simulink model "PubIfDecisionLSM_MDL"  (R2020b)
settings: configuration reference "DspaceConfig" (kept outside this file)
PostLoadFcn:
  | if any(exist('dsrtsu_mdlpostloadfcn', 'file') ~= 0), dsrtsu_mdlpostloadfcn('Execute', bdroot); end
InitFcn:
  | , if any(exist('rtifpga_mdlclblib', 'file') ~= 0), rtifpga_mdlclblib('Init', bdroot); end,
  | , if any(exist('dsmpb_private', 'file') ~= 0), dsmpb_private('dsmpb_mdlclblib', 'Init', bdroot); end,
values from neighbouring files (symbols this model uses):
  P_LSM_ALC_Enable = 0.0    [LSM_Parameter.sldd]
  P_LSM_AwayEdge_offset = 0.1    [LSM_Parameter.sldd]
  P_LSM_CentValidErr = 1.0    [LSM_Parameter.sldd]
  P_LSM_DOP_C0_EN_Limit = 0.8    [LSM_Parameter.sldd]
  P_LSM_DOP_C0_out_Limit = 2.0    [LSM_Parameter.sldd]
  P_LSM_DOP_C1_EN_Limit : value not decoded    [LSM_Parameter.sldd]
  P_LSM_DOP_C1_out_Limit : value not decoded    [LSM_Parameter.sldd]
  P_LSM_DOP_C1AndC2_Lim_X : value not decoded    [LSM_Parameter.sldd]
  P_LSM_DOP_C2_EN_Limit : value not decoded    [LSM_Parameter.sldd]
  P_LSM_DOP_C2_out_Limit : value not decoded    [LSM_Parameter.sldd]
  P_LSM_DOP_In_Pre2Dop_Dis = 1.0    [LSM_Parameter.sldd]
  P_LSM_DOP_Out_Pre2Dop_Dis = 2.0    [LSM_Parameter.sldd]
  P_LSM_DOP_PreDis_X : value not decoded    [LSM_Parameter.sldd]
  P_LSM_DOP_PreDis_Y : value not decoded    [LSM_Parameter.sldd]
  P_LSM_DOPEnableSW = 1.0    [LSM_Parameter.sldd]
  P_LSM_DOPValid_CheckTime = 0.06    [LSM_Parameter.sldd]
  P_LSM_DoubleLine_Curr2Cent_Dislimit = 0.5    [LSM_Parameter.sldd]
  P_LSM_DoubleLine_Dop2Cent_Dislimit = 0.5    [LSM_Parameter.sldd]
  P_LSM_DoubleLine_DOPOut_C1 : value not decoded    [LSM_Parameter.sldd]
  P_LSM_DoubleLine_Pre2Cent_Dislimit = 1.0    [LSM_Parameter.sldd]
  P_LSM_Error_Limit = 0.5    [LSM_Parameter.sldd]
  P_LSM_IFV2CenterAxis = 0.0    [LSM_Parameter.sldd]
  P_LSM_IFV2RearAxis = 0.0    [LSM_Parameter.sldd]
  P_LSM_Line2Edge_limit = 0.5    [LSM_Parameter.sldd]
  P_LSM_Line_Error = 0.1    [LSM_Parameter.sldd]
  P_LSM_LineSTD_Limit = 0.15    [LSM_Parameter.sldd]
  P_LSM_NOH_Switch = 0.0    [LSM_Parameter.sldd]
  P_LSM_OTL_C0_Factor = 1.0    [LSM_Parameter.sldd]
  P_LSM_OTL_C1_Factor = 0.5    [LSM_Parameter.sldd]
  P_LSM_OTL_C2_Factor = 0.5    [LSM_Parameter.sldd]
  P_LSM_Pre2OnlyLineDis = 5.0    [LSM_Parameter.sldd]
  P_LSM_Pre_t = 0.0    [LSM_Parameter.sldd]
  P_LSM_SingleLine_Cent2Edge_Dislimit = 100.0    [LSM_Parameter.sldd]
  P_LSM_SingleLine_Curr2Cent_Dislimit = 0.2    [LSM_Parameter.sldd]
  P_LSM_SingleLine_Dop2Cent_Dislimit = 0.2    [LSM_Parameter.sldd]
  P_LSM_SingleLine_DOPOut_C1 : value not decoded    [LSM_Parameter.sldd]
  P_LSM_SingleLine_Pre2Cent_Dislimit = 0.5    [LSM_Parameter.sldd]
  P_LSM_TJALimitSpd = 60.0    [LSM_Parameter.sldd]
undefined symbols (not defined in the file or in its folder): P_lCS_IFV2CenterAxis, P_LCS_IFV2RearAxis, P_LSM_EntryEdge_offset, P_LSM_EntryLnChngEnSwitch, P_LSM_EntryVanishDis, P_LSM_LinetLostTime, P_LSM_LineWijCal_C12, P_LSM_LineWijCal_C13, P_LSM_MapValid_ErrorSwitch, P_LSM_PosLineLcFac, P_LSM_SpdLim_Stub_Spd, P_LSM_SpdLim_StubLength, P_LSM_SpdTurnAlarm
libraries: simulink x324, TrueDurationTime x11
(part 22 of 25)

== stateflow chart PubIfDecisionLSM_MDL/Subsystem1/TargetLineCalc_20ms2/TargetLineCalc/Subsystem3/Subsystem/Chart1 ==
  state on
    state EntryStub1
      du:
      if roadClass==1
      PilotRoadSts=26;
      LSM_PilotSPL=0xff;
      PilotSPLDist=0xffff;
      else
      PilotRoadSts=33;
      LSM_PilotSPL=uint8(SpdChgMax);
      PilotSPLDist=uint16(ChgSpd_Dis);
      end
      state Name
        du:
        if CruiseTurn>0
        if EntryStubVanishTurn>0
        if LaneChangeEnable>0
        PilotTurnSwSts =turndir;
        else
        if Entry_dC0V>0
        PilotTurnSwSts =4;
        end
        if Entry_dC0V<0
        PilotTurnSwSts=5;
        end
        end
        else
        PilotTurnSwSts =turndir;
        end
        else
        if Entry_dC0V>0
        PilotTurnSwSts =4;
        end
        if Entry_dC0V<0
        PilotTurnSwSts=5;
        end
        end
      (default) -> on.EntryStub1.Name
    state CruiseValid2
      PilotRoadSts=18;
      LSM_PilotSPL=uint8(SpdChgMax);
      PilotSPLDist=uint16(ChgSpd_Dis);
      state init
        state Name
          PilotTurnSwSts =3;
        state init4
          PilotTurnSwSts =6;
        state init5
          PilotTurnSwSts =3;
        state init3
          PilotTurnSwSts =7;
        (default) -> on.CruiseValid2.init.Name
        on.CruiseValid2.init.Name -> on.CruiseValid2.init.init3 [order 3] : [FrbRight>0]
        on.CruiseValid2.init.init3 -> on.CruiseValid2.init.Name : [FrbRight==0]
        on.CruiseValid2.init.Name -> on.CruiseValid2.init.init4 [order 1] : [FrbLeft>0]
        on.CruiseValid2.init.init4 -> on.CruiseValid2.init.Name : [FrbLeft==0]
        on.CruiseValid2.init.Name -> on.CruiseValid2.init.init5 [order 2] : [OneLane>0]
        on.CruiseValid2.init.init5 -> on.CruiseValid2.init.Name : [OneLane==0]
      state Name2 [commented out]
        PilotTurnSwSts=turndir;
      state init1
        PilotTurnSwSts =1;
      state init2
        PilotTurnSwSts =2;
      (default) -> on.CruiseValid2.init
      on.CruiseValid2.init -> on.CruiseValid2.Name2 [commented out] : [Vanish_turnleft>0]
      on.CruiseValid2.Name2 -> on.CruiseValid2.init [commented out] : [Vanish_turnleft==0]
      on.CruiseValid2.init -> on.CruiseValid2.init1 [order 1] : [CruiseTurn>0&&...
          | TurnLeft>0]
      on.CruiseValid2.init1 -> on.CruiseValid2.init [order 1] : [CruiseTurn==0]
      on.CruiseValid2.init -> on.CruiseValid2.init2 [order 2] : [CruiseTurn>0&&...
          | TurnRight>0]
      on.CruiseValid2.init2 -> on.CruiseValid2.init [order 1] : [CruiseTurn==0]
      on.CruiseValid2.init2 -> on.CruiseValid2.init1 [order 2] : [TurnLeft>0]
      on.CruiseValid2.init1 -> on.CruiseValid2.init2 [order 2] : [TurnRight>0]
    state CruiseValid1
      PilotRoadSts=24;
      LSM_PilotSPL=0xff;
      PilotSPLDist=0xffff;
      state init
        state Name
          PilotTurnSwSts =3;
        state init4
          PilotTurnSwSts =6;
        state init5
          PilotTurnSwSts =3;
        state init3
          PilotTurnSwSts =7;
        (default) -> on.CruiseValid1.init.Name
        on.CruiseValid1.init.Name -> on.CruiseValid1.init.init3 [order 3] : [FrbRight>0]
        on.CruiseValid1.init.init3 -> on.CruiseValid1.init.Name : [FrbRight==0]
        on.CruiseValid1.init.Name -> on.CruiseValid1.init.init4 [order 1] : [FrbLeft>0]
        on.CruiseValid1.init.init4 -> on.CruiseValid1.init.Name : [FrbLeft==0]
        on.CruiseValid1.init.Name -> on.CruiseValid1.init.init5 [order 2] : [OneLane>0]
        on.CruiseValid1.init.init5 -> on.CruiseValid1.init.Name : [OneLane==0]
      state Name2 [commented out]
        PilotTurnSwSts=turndir;
      state init1
        PilotTurnSwSts =1;
      state init2
        PilotTurnSwSts =2;
      (default) -> on.CruiseValid1.init
      on.CruiseValid1.init -> on.CruiseValid1.Name2 [commented out] : [Vanish_turnleft>0]
      on.CruiseValid1.Name2 -> on.CruiseValid1.init [commented out] : [Vanish_turnleft==0]
      on.CruiseValid1.init -> on.CruiseValid1.init1 [order 2] : [CruiseTurn>0&&...
          | TurnLeft>0]
      on.CruiseValid1.init1 -> on.CruiseValid1.init [order 1] : [CruiseTurn==0]
      on.CruiseValid1.init -> on.CruiseValid1.init2 [order 1] : [CruiseTurn>0&&...
          | TurnRight>0]
      on.CruiseValid1.init2 -> on.CruiseValid1.init [order 1] : [CruiseTurn==0]
      on.CruiseValid1.init2 -> on.CruiseValid1.init1 [order 2] : [TurnLeft>0]
      on.CruiseValid1.init1 -> on.CruiseValid1.init2 [order 2] : [TurnRight>0]
    state CruiseValid
      PilotRoadSts=17;
      LSM_PilotSPL=0xff;
      PilotSPLDist=0xffff;
      state init
        state Name
          PilotTurnSwSts =0;
        state init4
          PilotTurnSwSts =6;
        state init5
          PilotTurnSwSts =3;
        state init3
          PilotTurnSwSts =7;
        (default) -> on.CruiseValid.init.Name
        on.CruiseValid.init.Name -> on.CruiseValid.init.init3 [order 3] : [FrbRight>0]
        on.CruiseValid.init.init3 -> on.CruiseValid.init.Name : [FrbRight==0]
        on.CruiseValid.init.Name -> on.CruiseValid.init.init4 [order 1] : [FrbLeft>0]
        on.CruiseValid.init.init4 -> on.CruiseValid.init.Name : [FrbLeft==0]
        on.CruiseValid.init.Name -> on.CruiseValid.init.init5 [order 2] : [OneLane>0]
        on.CruiseValid.init.init5 -> on.CruiseValid.init.Name : [OneLane==0]
      state Name2 [commented out]
        PilotTurnSwSts=turndir;
      state init1
        PilotTurnSwSts =1;
      state init2
        PilotTurnSwSts =2;
      on.CruiseValid.init -> on.CruiseValid.Name2 [commented out] : [Vanish_turnleft>0]
      (default) -> on.CruiseValid.init
      on.CruiseValid.Name2 -> on.CruiseValid.init [commented out] : [Vanish_turnleft==0]
      on.CruiseValid.init -> on.CruiseValid.init1 [order 1] : [CruiseTurn>0&&...
          | TurnLeft>0]
      on.CruiseValid.init1 -> on.CruiseValid.init [order 1] : [CruiseTurn==0]
      on.CruiseValid.init -> on.CruiseValid.init2 [order 2] : [CruiseTurn>0&&...
          | TurnRight>0]
      on.CruiseValid.init2 -> on.CruiseValid.init [order 1] : [CruiseTurn==0]
      on.CruiseValid.init2 -> on.CruiseValid.init1 [order 2] : [TurnLeft>0]
      on.CruiseValid.init1 -> on.CruiseValid.init2 [order 2] : [TurnRight>0]
    state EntryStub2
      PilotTurnSwSts =0;
      du:
      if roadClass==1
      PilotRoadSts=25;
      LSM_PilotSPL=0xff;
      PilotSPLDist=0xffff;
      else
      PilotRoadSts=32;
      LSM_PilotSPL=uint8(SpdChgMax);
      PilotSPLDist=uint16(ChgSpd_Dis);
      end
    state EntryTakeOver
      PilotRoadSts=31;
      LSM_PilotSPL=uint8(30);
      PilotSPLDist=uint16(0);
      PilotTurnSwSts =4;
    state StubValid
      state EntryStub3
        PilotTurnSwSts =turndir;
        PilotRoadSts=2;
        LSM_PilotSPL=uint8(SpdChgMax);
        PilotSPLDist=uint16(ChgSpd_Dis);
      state EntryStub4
        PilotTurnSwSts =turndir;
        PilotRoadSts=1;
        LSM_PilotSPL=uint8(SpdChgMax);
        PilotSPLDist=uint16(ChgSpd_Dis);
      state init
        PilotTurnSwSts =0;
        PilotRoadSts=0;
        LSM_PilotSPL=0xff;
        PilotSPLDist=0xffff;
      state EntryStub1
        PilotTurnSwSts =turndir;
        PilotRoadSts=2;
        LSM_PilotSPL=uint8(SpdChgMax);
        PilotSPLDist=uint16(ChgSpd_Dis);
      state EntryStub2
        PilotTurnSwSts =turndir;
        PilotRoadSts=1;
        LSM_PilotSPL=uint8(SpdChgMax);
        PilotSPLDist=uint16(ChgSpd_Dis);
      state LeftStub
        PilotTurnSwSts =turndir;
        PilotRoadSts=9;
        LSM_PilotSPL=0xff;
        PilotSPLDist=0xffff;
      state Name
        PilotTurnSwSts =turndir;
        PilotRoadSts=7;
        LSM_PilotSPL=0xff;
        PilotSPLDist=0xffff;
      state CruiseLeft
        PilotRoadSts=9;
        LSM_PilotSPL=uint8(StudLengthSpd);
        PilotSPLDist=uint16(f_distance);
        du:
        if f_distance<20
        PilotTurnSwSts=4;
        else
        PilotTurnSwSts=3;
        end
      state Name2
        PilotRoadSts=7;
        LSM_PilotSPL=uint8(StudLengthSpd);
        PilotSPLDist=uint16(f_distance);
        du:
        if f_distance<20
        PilotTurnSwSts=5;
        else
        PilotTurnSwSts=3;
        end
      state lExitStub3
        PilotTurnSwSts =turndir;
        PilotRoadSts=20;
        LSM_PilotSPL=uint8(SpdChgMax);
        PilotSPLDist=uint16(ChgSpd_Dis);
      state Name3
        PilotTurnSwSts =5;
        PilotRoadSts=8;
        LSM_PilotSPL=uint8(StudLengthSpd);
        PilotSPLDist=uint16(f_distance);
      state Name4
        PilotTurnSwSts =turndir;
        PilotRoadSts=20;
        LSM_PilotSPL=uint8(SpdChgMax);
        PilotSPLDist=uint16(ChgSpd_Dis);
      state lExitStub1
        PilotTurnSwSts =4;
        PilotRoadSts=10;
        LSM_PilotSPL=uint8(StudLengthSpd);
        PilotSPLDist=uint16(f_distance);
      state lExitStub2
        PilotTurnSwSts =4;
        PilotRoadSts=30;
        LSM_PilotSPL=uint8(SpdChgMax);
        PilotSPLDist=uint16(ChgSpd_Dis);
      state Name5
        PilotTurnSwSts =5;
        PilotRoadSts=19;
        LSM_PilotSPL=uint8(SpdChgMax);
        PilotSPLDist=uint16(ChgSpd_Dis);
      EntryStub4 -> EntryStub3 [order 1] : [EntryStub3>0]
      EntryStub3 -> EntryStub4 [order 1] : [EntryStub4>0]
      (default) -> on.StubValid.init
      on.StubValid.init -> EntryStub4 [order 4] : [EntryStub4>0]
      EntryStub4 -> on.StubValid.init [order 2] : [EntryStub3==0&&EntryStub4==0]
      on.StubValid.init -> EntryStub3 [order 2] : [EntryStub3>0]
      EntryStub3 -> on.StubValid.init [order 2] : [EntryStub3==0&&EntryStub4==0]
      on.StubValid.init -> on.StubValid.EntryStub1 [order 7] : [EntryStub1>0]
      on.StubValid.EntryStub1 -> on.StubValid.init [order 2] : [EntryStub1==0&&EntryStub2==0]
      on.StubValid.EntryStub1 -> on.StubValid.EntryStub2 [order 1] : [EntryStub2>0]
      on.StubValid.EntryStub2 -> on.StubValid.EntryStub1 [order 1] : [EntryStub1>0]
      on.StubValid.init -> on.StubValid.EntryStub2 [order 8] : [EntryStub2>0]
      on.StubValid.EntryStub2 -> on.StubValid.init [order 2] : [EntryStub1==0&&EntryStub2==0]
      (junction 434) -> on.StubValid.init
      on.StubValid.init -> (junction 601) [order 12] : [lExitStub2>0]
      (junction 453) -> on.StubValid.init
      on.StubValid.init -> CruiseLeft [order 5] : [CruiseLeft>0]
      CruiseLeft -> on.StubValid.init [order 3] : [CruiseLeft==0&&...
          | LeftStub==0&&...
          | rExitStub1==0]
      on.StubValid.init -> LeftStub [order 6] : [LeftStub>0]
      LeftStub -> on.StubValid.init [order 2] : [LeftStub==0&&CruiseLeft==0]
      on.StubValid.init -> lExitStub1 [order 10] : [lExitStub1>0]
      on.StubValid.init -> lExitStub3 [commented out] : [lExitStub3>0]
      lExitStub3 -> on.StubValid.init [order 3] : [lExitStub2==0&&...
          | lExitStub3==0&&...
          | lExitStub1==0]
      (junction 266) -> on.StubValid.init
      on.StubValid.init -> (junction 596) [order 11] : [rExitStub2>0]
      (junction 280) -> on.StubValid.init
      on.StubValid.init -> on.StubValid.Name2 [order 3] : [CruiseRight>0]
      on.StubValid.Name2 -> on.StubValid.init [order 3] : [CruiseRight==0&&...
          | RightStub==0&&...
          | rExitStub1==0]
      on.StubValid.init -> on.StubValid.Name [order 1] : [RightStub>0]
      on.StubValid.Name -> on.StubValid.init [order 2] : [RightStub==0&&CruiseRight==0]
      on.StubValid.init -> Name3 [order 9] : [rExitStub1>0]
      on.StubValid.init -> Name4 [commented out] : [rExitStub3>0]
      Name4 -> on.StubValid.init [order 3] : [rExitStub2==0&&...
          | rExitStub3==0&&...
          | rExitStub1==0]
      on.StubValid.Name -> on.StubValid.Name2 [order 1] : [CruiseRight>0]
      LeftStub -> CruiseLeft [order 1] : [CruiseLeft>0]
      on.StubValid.Name2 -> on.StubValid.Name [order 2] : [RightStub>0]
      CruiseLeft -> LeftStub [order 2] : [LeftStub>0]
      CruiseLeft -> lExitStub1 [order 1] : [lExitStub1>0]
      on.StubValid.Name2 -> Name3 [order 1] : [rExitStub1>0]
      Name3 -> Name4 [order 1] : [rExitStub3>0]
      lExitStub1 -> CruiseLeft [order 3] : [CruiseLeft>0]
      lExitStub1 -> lExitStub3 [order 1] : [lExitStub3>0]
      Name3 -> on.StubValid.Name2 [order 3] : [CruiseRight>0]
      Name4 -> Name3 [order 2] : [rExitStub1>0]
      lExitStub3 -> lExitStub1 [order 2] : [lExitStub1>0]
      lExitStub1 -> (junction 453) [order 4] : [CruiseLeft==0&&...
          | lExitStub1==0&&...
          | lExitStub3==0&&...
          | lExitStub2==0]
      Name3 -> (junction 280) [order 4] : [CruiseRight==0&&...
          | rExitStub1==0&&...
          | rExitStub3==0&&...
          | rExitStub2==0]
      lExitStub2 -> lExitStub3 [order 1] : [lExitStub3>0]
      lExitStub3 -> lExitStub2 [order 1] : [lExitStub2>0]
      Name3 -> Name5 [order 2] : [rExitStub2>0]
      Name5 -> Name3 [order 2] : [rExitStub1>0]
      Name4 -> Name5 [order 1] : [rExitStub2>0]
      Name5 -> Name4 [order 1] : [rExitStub3>0]
      lExitStub1 -> lExitStub2 [order 2] : [lExitStub2>0]
      lExitStub2 -> lExitStub1 [order 2] : [lExitStub1>0]
      (junction 596) -> Name5
      (junction 601) -> lExitStub2
      lExitStub2 -> (junction 434) [order 3] : [lExitStub2==0&&lExitStub3==0&&lExitStub1==0]
      Name5 -> (junction 266) [order 3] : [rExitStub2==0&&rExitStub3==0&&rExitStub1==0]
    state CruiseValid3
      PilotRoadSts=29;
      LSM_PilotSPL=0xff;
      PilotSPLDist=0xffff;
      state init
        state Name
          PilotTurnSwSts =3;
        state init4
          PilotTurnSwSts =6;
        state init5
          PilotTurnSwSts =3;
        state init3
          PilotTurnSwSts =7;
        (default) -> on.CruiseValid3.init.Name
        on.CruiseValid3.init.Name -> on.CruiseValid3.init.init3 [order 3] : [FrbRight>0]
        on.CruiseValid3.init.init3 -> on.CruiseValid3.init.Name : [FrbRight==0]
        on.CruiseValid3.init.Name -> on.CruiseValid3.init.init4 [order 1] : [FrbLeft>0]
        on.CruiseValid3.init.init4 -> on.CruiseValid3.init.Name : [FrbLeft==0]
        on.CruiseValid3.init.Name -> on.CruiseValid3.init.init5 [order 2] : [OneLane>0]
        on.CruiseValid3.init.init5 -> on.CruiseValid3.init.Name : [OneLane==0]
      state Name2 [commented out]
        PilotTurnSwSts=turndir;
      state init1
        PilotTurnSwSts =1;
      state init2
        PilotTurnSwSts =2;
      (default) -> on.CruiseValid3.init
      on.CruiseValid3.init -> on.CruiseValid3.Name2 [commented out] : [Vanish_turnleft>0]
      on.CruiseValid3.Name2 -> on.CruiseValid3.init [commented out] : [Vanish_turnleft==0]
      on.CruiseValid3.init -> on.CruiseValid3.init1 [order 2] : [CruiseTurn>0&&...
          | TurnLeft>0]
      on.CruiseValid3.init1 -> on.CruiseValid3.init [order 1] : [CruiseTurn==0]
      on.CruiseValid3.init -> on.CruiseValid3.init2 [order 1] : [CruiseTurn>0&&...
          | TurnRight>0]
      on.CruiseValid3.init2 -> on.CruiseValid3.init [order 1] : [CruiseTurn==0]
      on.CruiseValid3.init2 -> on.CruiseValid3.init1 [order 2] : [TurnLeft>0]
      on.CruiseValid3.init1 -> on.CruiseValid3.init2 [order 2] : [TurnRight>0]
    (junction 533) -> (junction 532)
    CruiseValid -> (junction 533) [order 3] : [RoadType==7]
    (junction 532) -> CruiseValid2
    (junction 527) -> (junction 528)
    (junction 528) -> CruiseValid
    CruiseValid2 -> (junction 527) [order 1] : [RoadType==1&&LSM_PilotNohExitDist>100]
    on.EntryStub1 -> CruiseValid [order 1] : [CruiseValid>0&&RoadType==1&&EntryStub5==0&&EntryStub6==0&&LSM_PilotNohExitDist>100]
    CruiseValid -> on.EntryStub1 [order 4] : [EntryStub5>0]
    CruiseValid1 -> CruiseValid2 [order 3] : [RoadType==7]
    CruiseValid -> CruiseValid1 [order 2] : [RoadType==2]
    on.EntryStub2 -> on.EntryStub1 [order 2] : [EntryStub5>0]
    on.EntryStub1 -> on.EntryStub2 [order 2] : [EntryStub6>0]
    on.EntryStub1 -> EntryTakeOver [order 4] : [EntryStub5_takeover>0&&...
        | Entry_dC0V>0]
    CruiseValid2 -> CruiseValid1 [order 3] : [RoadType==2]
    CruiseValid1 -> CruiseValid [order 2] : [RoadType==1&&LSM_PilotNohExitDist>100]
    CruiseValid -> on.EntryStub2 [order 5] : [EntryStub6>0]
    on.EntryStub2 -> CruiseValid [order 1] : [CruiseValid>0&&...
        | RoadType==1&&...
        | EntryStub5==0&&...
        | EntryStub6==0&&LSM_PilotNohExitDist>100]
    CruiseValid2 -> StubValid [order 2] : [StubValid>0]
    StubValid -> CruiseValid2 [order 5] : [CruiseValid>0&&RoadType==7&&EntryStub5==0&&EntryStub6==0&&roadClass==0]
    StubValid -> on.EntryStub2 [order 3] : [EntryStub6>0]
    on.EntryStub2 -> StubValid [order 3] : [EntryStub5==0&&EntryStub6==0]
    CruiseValid -> StubValid [order 1] : [StubValid>0]
    StubValid -> CruiseValid [order 1] : [CruiseValid>0&&RoadType==1&&EntryStub5==0&&EntryStub6==0&&LSM_PilotNohExitDist>100]
    CruiseValid1 -> StubValid [order 1] : [StubValid>0]
    StubValid -> CruiseValid1 [order 4] : [CruiseValid>0&&RoadType==2&&EntryStub5==0&&EntryStub6==0]
    EntryTakeOver -> StubValid : [EntryStub5_takeover==0]
    StubValid -> on.EntryStub1 [order 2] : [EntryStub5>0]
    on.EntryStub1 -> StubValid [order 3] : [EntryStub5==0&&EntryStub6==0]
    (default) -> StubValid
    StubValid -> CruiseValid3 [order 6] : [RoadType~=7&&RoadType~=1&&...
        | RoadType~=2&&CruiseValid>0]
    CruiseValid3 -> StubValid : [StubValid>0||RoadType==1||...
        | RoadType==2||RoadType==7]
  state off1
    PilotTurnSwSts =3;
    PilotRoadSts =0;
    LSM_PilotSPL=0xff;
    PilotSPLDist=0xffff;
  state HWA
    PilotTurnSwSts =0;
    PilotRoadSts =0;
    LSM_PilotSPL=0xff;
    PilotSPLDist=0xffff;
  (default) -> off1
  off1 -> on [order 1] : [(i_mapvalid==2||i_mapvalid==3)&&...
      | i_on_nav_path==1&&...
      | NOH_Sts>2]
  on -> off1 [order 1] : [NOH_Sts<3||...
      | i_mapvalid==0||...
      | ((i_mapvalid==1||...
      | (i_mapvalid==2&&i_on_nav_path~=1)||...
      | (i_mapvalid==3&&i_on_nav_path~=1)||...
      | i_mapvalid==4||...
      | i_mapvalid==5)&&...
      | RoadType~=1)]
  off1 -> HWA [order 2] : [(i_mapvalid==1||...
      | (i_mapvalid==2&&i_on_nav_path~=1)||...
      | (i_mapvalid==3&&i_on_nav_path~=1)||...
      | i_mapvalid==4||...
      | i_mapvalid==5)&&...
      | RoadType==1]
  HWA -> off1 [order 2] : [i_mapvalid==0||RoadType~=1]
  HWA -> on [order 1] : [(i_mapvalid==2||i_mapvalid==3)&&...
      | i_on_nav_path==1&&...
      | NOH_Sts>2]
  on -> HWA [order 2] : [(i_mapvalid==1||...
      | (i_mapvalid==2&&i_on_nav_path~=1)||...
      | (i_mapvalid==3&&i_on_nav_path~=1)||...
      | i_mapvalid==4||...
      | i_mapvalid==5)&&...
      | RoadType==1]
  data: StubValid input boolean size=1; RightStub input boolean size=1; RoadType input uint8 size=1; PilotRoadSts output uint8 size=1; PilotTurnSwSts output uint8 size=1; LeftStub input boolean size=1; CruiseValid input boolean size=1; TurnLeft input boolean size=1; TurnRight input boolean size=1; Vanish_turnleft input uint8 size=1; EntryStub1 input boolean size=1; rExitStub1 input boolean size=1; rExitStub2 input boolean size=1; i_mapvalid input uint8 size=1; i_on_nav_path input uint8 size=1; CruiseLeft input boolean size=1; CruiseRight input boolean size=1; f_distance input single size=1; LSM_PilotSPL output uint8 size=1; PilotSPLDist output uint16 size=1; CruiseTurn input boolean size=1; EntryStub2 input boolean size=1; lExitStub1 input boolean size=1; lExitStub2 input boolean size=1; lExitStub3 input boolean size=1; rExitStub3 input boolean size=1; FrbLeft input boolean size=1; FrbRight input boolean size=1; OneLane input boolean size=1; EntryStub3 input; EntryStub4 input; EntryStub5 input; EntryStub6 input; EntryStub5_takeover input; turndir input; roadClass input; LSM_PilotNohExitDist input; i local; Entry_dC0V input; StudLengthSpd input; EntryStubVanishTurn input; LaneChangeEnable input; NOH_Sts input; ChgSpd_Dis input; SpdChgMax input

== stateflow chart PubIfDecisionLSM_MDL/Subsystem1/TargetLineCalc_20ms2/TargetLineCalc/Subsystem3/Subsystem/Chart2 ==
  state Name
    y=PilotRoadSts;
  state Name1
    y=uint8(0);
  (default) -> Name
  Name -> Name1 : [PilotRoadSts==17&&...
      | PilotRoadStsK~=17&&...
      | LSM_PilotNohExitDist<100]
  Name1 -> Name : [LSM_PilotNohExitDist>=100]
  data: LSM_PilotNohExitDist input; PilotRoadSts input uint8; PilotRoadStsK input uint8; y output uint8

== stateflow chart PubIfDecisionLSM_MDL/Subsystem1/TargetLineCalc_20ms2/TargetLineCalc/Subsystem3/Subsystem/Chart3 ==
  state Name
    y=PilotSts;
  state Name1
    en:
    y=uint8(0);
    i=uint8(0);
    Dis=single(0);
    du:
    i=i+1;
    Dis=Dis+vehSpd*0.02;
  (default) -> Name
  Name -> Name1 : [(NOH_Sts~=3&&NOH_StsK==3)||...
      | (PilotSts==0&&PilotStsK~=0)]
  Name1 -> Name : [i>150&&Dis>100]
  data: y output uint8; PilotSts input; NOH_Sts input; NOH_StsK input; PilotStsK input; vehSpd input; i local; Dis local single

== matlab function PubIfDecisionLSM_MDL/Subsystem1/TargetLineCalc_20ms2/TargetLineCalc/Subsystem3/Subsystem/MATLAB Function ==
  data: NOH_Valid input boolean size=1; PilotSts output uint8 size=1; RoadType input uint8 size=1; LSM_PilotNohExitDist input; rExitStub4_takeover input; lExitStub4_takeover input; EntryStub5_takeover input; Vanish_turnleft_takeover input; ForbidActive input
function PilotSts = fcn(NOH_Valid,RoadType,LSM_PilotNohExitDist,rExitStub4_takeover,lExitStub4_takeover,...
    EntryStub5_takeover,Vanish_turnleft_takeover,ForbidActive)
PilotSts=uint8(0);
if NOH_Valid == 1 && LSM_PilotNohExitDist>50 && ForbidActive==0
    if RoadType == 1
        PilotSts = uint8(1); %NOH-HW Mode
    end
    if RoadType == 2
        PilotSts = uint8(4); %NOH-City Mode
    end
    if RoadType ~=1 && RoadType ~=2
        PilotSts = uint8(2); %NOH-Ramp Mode
    end
%     if rExitStub4_takeover>0 || lExitStub4_takeover>0 || EntryStub5_takeover>0 || Vanish_turnleft_takeover>0
%         PilotSts = uint8(3); %NOH-TakeOver
%     end
end

== matlab function PubIfDecisionLSM_MDL/Subsystem1/TargetLineCalc_20ms2/TargetLineCalc/Subsystem3/Subsystem/Subsystem/MATLAB Function ==
  data: count input; PilotNohExitDist output; NoPUCR output; startDis input; type input; NoPUCR_Dis output
function [PilotNohExitDist,NoPUCR,NoPUCR_Dis] = fcn(count,startDis,type)
PilotNohExitDist = 0xffff;
NoPUCR_Dis = 0xffff;
NoPUCR=uint8(0);
% for i=1:count
%     if type(i)== 18446744073709551612 
%         PilotNohExitDist = startDis(i);
%     end
%     if type(i)== 18446744073709551613 || type(i)== 18446744073709551614
%         if (endDis(i)-startDis(i))> 200
% ODD_valid = uint8(zeros(5,1));
if count>0
    for i=1:count
        if  type(i)~= 18446744073709551614 && type(i)~= 4096 && type(i)~= 8 
%         if bitand(type(i),4,'uint64')==1 || type(i)==18446744073709551612 || type(i)==18446744073709551613||type(i)== 18446744073709551614
            PilotNohExitDist = uint16(startDis(i));
            break;
        end
        if type(i) == 18446744073709551614
            NoPUCR=uint8(1);
            NoPUCR_Dis=uint16(startDis(i));
        end
    end
end

== matlab function PubIfDecisionLSM_MDL/Subsystem1/TargetLineCalc_20ms2/TargetLineCalc/Subsystem3/Subsystem1/MATLAB Function ==
  data: i_mapvalid_out output uint8; i_on_nav_path_out output uint8; RoadType_out output; count output uint16; time_trigger output uint8; RoadStore output uint8; i_mapvalid_store output uint8; i_on_nav_path_store output uint8; f_distance_store output single; i_mapvalid input uint8; i_mapvalidK input uint8; i_on_nav_path input uint8; i_on_nav_pathK input uint8; RoadType input; RoadTypeK input uint8; f_distanceK input single; countK input uint16; timing_triggerK input uint8; RoadStoreK input uint8; i_mapvalid_storeK input uint8; i_on_nav_path_storeK input uint8; f_distance_storeK input single
function [i_mapvalid_out,i_on_nav_path_out,RoadType_out,count,time_trigger,RoadStore,i_mapvalid_store,i_on_nav_path_store,f_distance_store] = fcn(i_mapvalid,i_mapvalidK,i_on_nav_path,i_on_nav_pathK,...
    RoadType,RoadTypeK,f_distanceK,countK,timing_triggerK,RoadStoreK,i_mapvalid_storeK,i_on_nav_path_storeK,f_distance_storeK)
time_trigger = timing_triggerK;
RoadStore =RoadStoreK;
i_mapvalid_store = i_mapvalid_storeK;
i_on_nav_path_store = i_on_nav_path_storeK;
f_distance_store = f_distance_storeK;
if (i_mapvalid~=2&&i_mapvalid~=3) && (i_mapvalidK==2||i_mapvalidK==3)
    timing_trigger = uint8(1);
else
    timing_trigger = uint8(0);
end
[time3,time5,time10,count]=clculagraph(timing_trigger,countK);

if (i_mapvalid~=2&&i_mapvalid~=3) && (i_mapvalidK==2||i_mapvalidK==3)
    i_mapvalid_store =  i_mapvalidK;
    i_on_nav_path_store = i_on_nav_pathK;
    f_distance_store = f_distanceK;
    RoadStore = RoadTypeK;
    
end
if  i_mapvalid~=2&&i_mapvalid~=3
    if ((f_distance_store>200 || f_distance_store == 0) && (RoadStore==1 && time10==0) || (RoadStore~=1 && time5==0))||...
           ((f_distance_store<=200 && f_distance_store > 0) && time3==0 )
       i_mapvalid_out = i_mapvalid_store;
       i_on_nav_path_out = i_on_nav_path_store;
       RoadType_out = RoadStore;
    else
       i_mapvalid_out = i_mapvalid;
       i_on_nav_path_out = i_on_nav_path; 
       RoadType_out = RoadType;
    end
else
       i_mapvalid_out = i_mapvalid;
       i_on_nav_path_out = i_on_nav_path; 
       RoadType_out = RoadType;
end
end

function [time3,time5,time10,cnt]=clculagraph(event,cntk)
time3 = uint8(0);
time5 = uint8(0);
time10 = uint8(0);
if event == 1
     cntk = uint16(150);
end
if cntk > 0
     cntk = cntk - 1;
end
if cntk < 100 
    time3 = uint8(1);
end
if cntk < 50 
    time5 = uint8(1);
end
if cntk == 0 
    time10 = uint8(1);
end
cnt = cntk;
end

== stateflow chart PubIfDecisionLSM_MDL/Subsystem1/TargetLineCalc_20ms2/TargetLineCalc/Subsystem3/Subsystem1/Subsystem/Chart ==
  state Name
    y=nav_path;
  state Name1
    y=uint8(1);
  (default) -> Name
  Name -> Name1 : [nav_path==0&&nav_pathK==1&&...
      | NoPUCR==0]
  Name1 -> Name : [nav_path==0&&...
      | NoPUCR==1]
  data: NoPUCR input; nav_path input; nav_pathK input; y output

== matlab function PubIfDecisionLSM_MDL/Subsystem1/TargetLineCalc_20ms2/TargetLineCalc/Subsystem3/Subsystem1/Subsystem/MATLAB Function1 ==
  data: u input; y output; uK input; count output; countK input uint8
function [y,count] = fcn(u,uK,countK)
count=max(countK-uint8(1),uint8(0));
if u==0&&uK==1
    count=uint8(150);
end
if count>0
    y=uint8(1);
else
    y=u;
end

== matlab function PubIfDecisionLSM_MDL/Subsystem1/TargetLineCalc_20ms2/TargetLineCalc/Subsystem3/Subsystem2/MATLAB Function ==
  data: nLaneID input uint8 size=1; i_rec_lanes input uint8 size=8; Forbid_TurnRight output boolean size=1; Forbid_TurnLeft output boolean size=1; OneLane output boolean size=1; i_rec_lanes_num input
function [Forbid_TurnRight,Forbid_TurnLeft,OneLane] = fcn(nLaneID,i_rec_lanes,i_rec_lanes_num)

Forbid_TurnRight = false;
Forbid_TurnLeft = false;
OneLane = false;
m=uint8(1);
if i_rec_lanes_num == 1
    if nLaneID==i_rec_lanes(1)
        OneLane = true;
    end
end
if i_rec_lanes_num > 1 
    if i_rec_lanes(1)>1 && nLaneID==i_rec_lanes(1)
        Forbid_TurnLeft = true;
    end

    for i=uint8(1):length(i_rec_lanes)
        if i_rec_lanes(i)>0
            m=i;
        end
    end

    if nLaneID == i_rec_lanes(m)
        Forbid_TurnRight = true;
    end
end

== matlab function PubIfDecisionLSM_MDL/Subsystem1/TargetLineCalc_20ms2/TargetLineCalc/Subsystem3/Subsystem2/MATLAB Function1 ==
  data: rightLane_valid input; rightLane_type input; turndir output; leftLane_valid input; leftLane_type input; curr_vanish_valid input; curr_vanish_pt_dis input; currentLane_type input; roadClass output uint8; left_vanish_valid input; left_vanish_pt_dis input; right_vanish_valid input; right_vanish_pt_dis input; DecSpd output; currentLane_valid input; ForbidActive output
function [turndir,roadClass,DecSpd,ForbidActive] = fcn(rightLane_valid, rightLane_type,leftLane_valid,leftLane_type,curr_vanish_valid,...
    curr_vanish_pt_dis,currentLane_type,left_vanish_valid,left_vanish_pt_dis,right_vanish_valid,right_vanish_pt_dis,currentLane_valid)
turndir = uint8(0);
roadClass = uint8(0);
DecSpd=uint8(0);
ForbidActive=uint8(0);
if curr_vanish_valid == 1
    if leftLane_valid == 1 && leftLane_type ~=5 && (left_vanish_valid==0||(left_vanish_valid==1&&(left_vanish_pt_dis>curr_vanish_pt_dis)))
        turndir = uint8(1);
        if leftLane_type == 1
            roadClass = uint8(1); %%高速
        else
            roadClass = uint8(0); %%匝道
        end
    else
        if rightLane_valid == 1 && rightLane_type ~=5 && (right_vanish_valid==0||(right_vanish_valid==1&&(right_vanish_pt_dis>curr_vanish_pt_dis)))
            turndir = uint8(2);
            if rightLane_type == 1
                roadClass = uint8(1); %%高速
            else
                roadClass = uint8(0); %%匝道
            end
        end
    end
    if curr_vanish_pt_dis<80 
        DecSpd=uint8(1);
    end
    
else
    if currentLane_type == 1 ||(rightLane_valid==1&&rightLane_type==1)||(leftLane_valid==1&&leftLane_type == 1)
        roadClass = uint8(1); %%高速
    else
        roadClass = uint8(0); %%匝道
    end
end

if currentLane_valid==1 && currentLane_type==5
    ForbidActive=uint8(1);
end

== matlab function PubIfDecisionLSM_MDL/Subsystem1/TargetLineCalc_20ms2/TargetLineCalc/Subsystem3/Subsystem2/MATLAB Function2 ==
  data: nLaneNum input; y output uint8; nLaneID input; en_direction input; PilotRoadSts input
function y = fcn(nLaneNum,nLaneID,en_direction,PilotRoadSts)
y=uint8(0);
if en_direction==2&&PilotRoadSts==7&&nLaneNum~=0
    y=abs(nLaneNum-nLaneID);
end
if en_direction==1&&PilotRoadSts==7&&nLaneNum~=0
    y=abs(nLaneNum-nLaneID);
end

== matlab function PubIfDecisionLSM_MDL/Subsystem1/TargetLineCalc_20ms2/TargetLineCalc/Subsystem3/Subsystem2/MATLAB Function3 ==
  data: i_rec_lanes input; y output
function y = fcn(i_rec_lanes)
y =  uint8(0); 
for i=1:8
    if i_rec_lanes(i)~=0
        y = uint8(1);  
        break;
    end 
end

== matlab function PubIfDecisionLSM_MDL/Subsystem1/TargetLineCalc_20ms2/TargetLineCalc/Subsystem3/Subsystem2/MATLAB Function4 ==
  data: rightLane_valid input; y output uint8; leftLane_valid input; curr_vanish_valid input; curr_vanish_pt_dis input; left_vanish_valid input; left_vanish_pt_dis input; right_vanish_valid input; right_vanish_pt_dis input
function y = fcn(rightLane_valid,leftLane_valid,curr_vanish_valid,...
    curr_vanish_pt_dis, left_vanish_valid,left_vanish_pt_dis,right_vanish_valid,right_vanish_pt_dis)
y = uint8(0);
if curr_vanish_valid == 1
    if (leftLane_valid == 1  && (left_vanish_valid==0||(left_vanish_valid==1&&(left_vanish_pt_dis>curr_vanish_pt_dis))))||...
            (rightLane_valid == 1 && (right_vanish_valid==0||(right_vanish_valid==1&&(right_vanish_pt_dis>curr_vanish_pt_dis))))
            y = uint8(1);
    end
end

== matlab function PubIfDecisionLSM_MDL/Subsystem1/TargetLineCalc_20ms2/TargetLineCalc/Subsystem3/Subsystem2/MATLAB Function5 ==
  data: b_vanish_valid input; VanishLaneTkOverValid output boolean; b_vanish_validK input; f_vanish_pt_dis input; VanishLaneTkOverValidK input boolean
function VanishLaneTkOverValid = fcn(b_vanish_valid,b_vanish_validK,f_vanish_pt_dis,VanishLaneTkOverValidK)
VanishLaneTkOverValid=VanishLaneTkOverValidK;
if b_vanish_valid==1&&b_vanish_validK==0&&f_vanish_pt_dis>100
    VanishLaneTkOverValid=true;
end
if b_vanish_valid==0
    VanishLaneTkOverValid=false;
end

== matlab function PubIfDecisionLSM_MDL/Subsystem1/TargetLineCalc_20ms2/TargetLineCalc/Subsystem3/Subsystem2/Subsystem/MATLAB Function4 ==
  data: u input uint8; y output uint8; uK input uint8; i output uint8; iK input uint8
function [y,i] = fcn(u,uK,iK)
i=max(iK-uint8(1),uint8(0));
if u==0&&uK>0
    i=uint8(50);
end
if i>0
    y=uint8(1);
else
    y=u;
end

== matlab function PubIfDecisionLSM_MDL/Subsystem1/TargetLineCalc_20ms2/TargetLineCalc/Subsystem3/Subsystem2/Subsystem1/MATLAB Function4 ==
  data: u input uint8; y output uint8; uK input uint8; i output uint8; iK input uint8
function [y,i] = fcn(u,uK,iK)
i=max(iK-uint8(1),uint8(0));
if u==0&&uK>0
    i=uint8(50);
end
if i>0
    y=uint8(1);
else
    y=u;
end

== matlab function PubIfDecisionLSM_MDL/Subsystem1/TargetLineCalc_20ms2/TargetLineCalc/Subsystem3/Subsystem2/Subsystem17/MATLAB Function1 ==
  data: b_is_available input; b_is_availableK input; enStubExist output uint8; Entry_bIsLineExist input; Entry_bIsLineExistK input; enStubExistK input uint8
function enStubExist = fcn(b_is_available,b_is_availableK,Entry_bIsLineExist,Entry_bIsLineExistK,enStubExistK)
enStubExist = enStubExistK;
if (b_is_available==1 && Entry_bIsLineExist==2) && (b_is_availableK==0 && Entry_bIsLineExistK==2 )
    enStubExist =  uint8(1);
end
if Entry_bIsLineExist < 2
    enStubExist = uint8(0);
end

== matlab function PubIfDecisionLSM_MDL/Subsystem1/TargetLineCalc_20ms2/TargetLineCalc/Subsystem3/Subsystem2/Subsystem2/MATLAB Function14 ==
  data: laneValid input boolean; laneValidK input boolean; u input; uK input; y output uint8; countK1 input uint8; count1 output uint8; y_storeK input uint8; y_store output uint8; timeValidK1 input uint8; countK2 input uint8; timeValid1 output uint8; timeValidK2 input uint8; count2 output uint8; timeValid2 output uint8
function [y,count1,y_store,timeValid1,count2,timeValid2] = fcn(laneValid,laneValidK,u,uK,countK1,y_storeK,timeValidK1,countK2,timeValidK2)

count1 = countK1;
count2 = countK2;
timeTrigger1 = uint8(0);
timeTrigger2 = uint8(0);
y_store = y_storeK;
timeValid1 = timeValidK1;
timeValid2 = timeValidK2;

if laneValid >0 && u<=2 && u>=-2
    y_temp = uint8(0);
else
    y_temp = uint8(1);
end

if laneValidK > 0
    if count2 == 0 && (uK>2 || uK<-2) && (u<=2 && u>=-2)
        timeTrigger1 = uint8(1);
        y_store = uint8(1);
    end
    if count1 == 0 && (uK<=2 && uK>=-2) && (u>2 || u<-2)
        timeTrigger2 = uint8(1);
        y_store = uint8(0);
    end
    [timeValid1,count1] = clculation(timeTrigger1,countK1,timeValidK1);
    [timeValid2,count2] = clculation(timeTrigger2,countK1,timeValidK2);

    if timeValid1>0 || timeValid2>0
        y = y_store;
    else
        y = y_temp;
    end
else
    y = y_temp;
end


function [m,cnt] = clculation(trigg,cntK,mK)
m=mK;
if trigg > 0
    cntK = uint8(10);
end
if cntK > 0
    cntK = cntK - 1;
    m = uint8(1);
end
if cntK == 0
    m = uint8(0);
end
cnt=cntK;

== stateflow chart PubIfDecisionLSM_MDL/Subsystem1/TargetLineCalc_20ms2/TargetLineCalc/Subsystem3/Subsystem4/Chart ==
  state Name
    NOH_HMI_Voice=0;
  state Name1
    state Name1
      NOH_HMI_Voice=1;%提醒即将进入匝道（汇出）
      en:i=0;
      du:i=i+1;
    state Name2
      NOH_HMI_Voice=0;
    state Name3
      %提醒手动变道（汇出，走不到最右侧）
      state Name
        NOH_HMI_Voice=2;
        en:m=0;
        du:m=m+1;
      state Name1
        NOH_HMI_Voice=0;
        en:n=0;
        du:n=n+1;
      (default) -> Name1.Name3.Name
      Name1.Name3.Name -> Name1.Name3.Name1 : [m>150]
      Name1.Name3.Name1 -> Name1.Name3.Name : [n>50]
    state Name4
      %提醒请手动进入匝道（汇出，走不上汇出线）
      state Name9
        NOH_HMI_Voice=3;
        en:m=0;
        du:m=m+1;
      state Name8
        NOH_HMI_Voice=0;
        en:n=0;
        du:n=n+1;
      (default) -> Name1.Name4.Name9
      Name1.Name4.Name9 -> Name1.Name4.Name8 : [m>150]
      Name1.Name4.Name8 -> Name1.Name4.Name9 : [n>50]
    (default) -> Name1.Name1
    Name1.Name1 -> Name1.Name2 : [i>150]
    Name1.Name4 -> Name1.Name2 [order 2] : [ExitStub4_takeover==0&&...
        | NoPUCR==0]
    Name1.Name2 -> Name1.Name4 [order 2] : [ExitStub4_takeover>0||...
        | (NoPUCR_Dis<400&&...
        | NoPUCR_Dis>0&&...
        | NoPUCR>0)]
    Name1.Name2 -> Name1.Name3 [order 1] : [exitTakeOverValid>0||...
        | PilotRoadSts==20]
    Name1.Name3 -> Name1.Name2 [order 2] : [exitTakeOverValid==0&&...
        | PilotRoadSts~=20]
    Name1.Name3 -> Name1.Name4 [order 1] : [ExitStub4_takeover>0]
    Name1.Name4 -> Name1.Name3 [order 1] : [exitTakeOverValid>0||...
        | PilotRoadSts==20]
  state Name2
    state Name1
      NOH_HMI_Voice=1;%提醒即将进入匝道（汇出）
      en:i=0;
      du:i=i+1;
    state Name2
      NOH_HMI_Voice=0;
    state Name3
      %提醒手动变道（汇出，走不到最右侧）
      state Name
        NOH_HMI_Voice=2;
        en:m=0;
        du:m=m+1;
      state Name1
        NOH_HMI_Voice=0;
        en:n=0;
        du:n=n+1;
      (default) -> Name2.Name3.Name
      Name2.Name3.Name -> Name2.Name3.Name1 : [m>150]
      Name2.Name3.Name1 -> Name2.Name3.Name : [n>50]
    state Name4
      %提醒请手动进入匝道（汇出，走不上汇出线）
      state Name9
        NOH_HMI_Voice=3;
        en:m=0;
        du:m=m+1;
      state Name8
        NOH_HMI_Voice=0;
        en:n=0;
        du:n=n+1;
      (default) -> Name2.Name4.Name9
      Name2.Name4.Name9 -> Name2.Name4.Name8 : [m>150]
      Name2.Name4.Name8 -> Name2.Name4.Name9 : [n>50]
    (default) -> Name2.Name1
    Name2.Name1 -> Name2.Name2 : [i>150]
    Name2.Name4 -> Name2.Name2 [order 2] : [ExitStub4_takeover==0&&...
        | NoPUCR==0]
    Name2.Name2 -> Name2.Name4 [order 2] : [ExitStub4_takeover>0||...
        | (NoPUCR_Dis<400&&...
        | NoPUCR_Dis>0&&...
        | NoPUCR>0)]
    Name2.Name2 -> Name2.Name3 [order 1] : [exitTakeOverValid>0||...
        | PilotRoadSts==20]
    Name2.Name3 -> Name2.Name2 [order 2] : [exitTakeOverValid==0&&...
        | PilotRoadSts~=20]
    Name2.Name3 -> Name2.Name4 [order 1] : [ExitStub4_takeover>0]
    Name2.Name4 -> Name2.Name3 [order 1] : [exitTakeOverValid>0||...
        | PilotRoadSts==20]
  state Name3
    %提醒手动汇入
    state Name8
      NOH_HMI_Voice=4;
      en:m=0;
      du:m=m+1;
    state Name1
      NOH_HMI_Voice=0;
      en:n=0;
      du:n=n+1;
    (default) -> Name3.Name8
    Name3.Name8 -> Name3.Name1 : [m>150]
    Name3.Name1 -> Name3.Name8 : [n>50]
  state Name4
    NOH_HMI_Voice=5;
    %更换到快速车道
    en:i=0;
    du:i=i+1;
  state Name5
    NOH_HMI_Voice=6;
    %已进入匝道，请注意前方路况
    en:i=0;
    du:i=i+1;
  state Name7
    NOH_HMI_Voice=8;
    %当前车道线不清晰，请注意驾驶
  state Name6
    NOH_HMI_Voice=7;
    %前方汇入，请注意侧方车辆
  (default) -> Name
  Name -> Name1 [order 1] : [en_direction==2]
  Name1 -> Name : [en_direction~=2]
  Name -> Name2 [order 4] : [en_direction==1]
  Name2 -> Name : [en_direction~=1]
  Name -> Name3 [order 3] : [((PilotRoadSts==26||PilotRoadSts==33)&&...
      | f_vanish_pt_dis<=EnVanDis&&...
      | b_vanish_valid>0&&HWASts~=5&&HWASts~=6)]
  Name3 -> Name : [(PilotRoadSts~=26&&PilotRoadSts~=33)||...
      | b_vanish_valid<1]
  Name -> Name4 [order 5] : [changeVoice==1]
  Name4 -> Name : [changeVoice==0&&i>150]
  Name -> Name5 [order 2] : [PilotRoadStsK==19&&...
      | PilotRoadSts~=19]
  Name5 -> Name : [i>150]
  Name -> Name6 [order 6] : [(en_direction==5&&...
      | f_distance<=80&&...
      | f_distance>0)||...
      | (en_direction==3&&...
      | f_distance<=80&&...
      | f_distance>0&&...
      | LaneNum<=2&&...
      | LaneNum>0)]
  Name6 -> Name : [(en_direction~=5&&...
      | en_direction~=3)||...
      | f_distance>80]
  Name -> Name7 [order 7] : [Double_Line_Lost>0]
  Name7 -> Name : [Double_Line_Lost==0]
  data: PilotRoadSts input; en_direction input; f_vanish_pt_dis input; i local; NOH_HMI_Voice output; changeVoice input; b_vanish_valid input; exitTakeOverValid input uint8; m local; n local; PilotRoadStsK input; ExitStub4_takeover input; f_distance input; Double_Line_Lost input; LaneNum input; NoPUCR input; NoPUCR_Dis input; EnVanDis input; HWASts input

== matlab function PubIfDecisionLSM_MDL/Subsystem1/TargetLineCalc_20ms2/TargetLineCalc/TJA2NOA ==
  data: TJALineValid input boolean size=1; HWALineValid output boolean size=1; TJALineA3 input single size=1; TJALineA2 input single size=1; TJALineA1 input single size=1; TJALineA0 input single size=1; TJALineRange input single size=1; HWALineC3 output single size=1; HWALineC2 output single size=1; HWALineC1 output single size=1; HWALineC0 output single size=1; HWARange output single size=1; HWALineC0K1 input
function [HWALineValid,HWALineC3,HWALineC2,HWALineC1,HWALineC0,HWARange] =...
    fcn(TJALineValid,TJALineA3,TJALineA2,...
    TJALineA1,TJALineA0,TJALineRange,HWALineC0K1)
HWALineValid = TJALineValid;
HWALineC3 = TJALineA3;
HWALineC2 = TJALineA2;
HWALineC1 = TJALineA1;
if abs(TJALineA0-HWALineC0K1)>1||abs(TJALineA0-HWALineC0K1)<0.05
    HWALineC0 = TJALineA0;
else
    HWALineC0 = 0.05*(TJALineA0-HWALineC0K1)+HWALineC0K1;
end
HWARange = TJALineRange;
% Wait_counter = max(uint8(0),Wait_counterK1-1);
% if TJALineValid==1&&TJALineValidK1==1
%     Y1K1 = TJALineA0K1+TJALineA1K1*Pre_dis+TJALineA2K1*Pre_dis^2+TJALineA3K1*Pre_dis^3;
%     Y1 = TJALineA0+TJALineA1*Pre_dis+TJALineA2*Pre_dis^2+TJALineA3*Pre_dis^3;
%     Error = Y1-Y1K1;
%     if abs(Error)<Error_limit
%         HWALineValid = TJALineValid;
%         HWALineC3 = TJALineA3;
%         HWALineC2 = TJALineA2;
%         HWALineC1 = TJALineA1;
%         HWALineC0 = TJALineA0;
%         HWARange = TJALineRange;
%     else
%         Wait_counter = uint8(100);
%     end
% end
% if Wait_counter==0
%     HWALineValid = TJALineValid;
%     HWALineC3 = TJALineA3;
%     HWALineC2 = TJALineA2;
%     HWALineC1 = TJALineA1;
%     HWALineC0 = TJALineA0;
%     HWARange = TJALineRange;
% end

== matlab function PubIfDecisionLSM_MDL/Subsystem1/TargetLineCalc_20ms2/TargetLineCalc/Tracker ==
  data: LeftOffset_b output boolean size=1; RightOffset_b output boolean size=1; LineUpdate input boolean size=1; LineConf input uint8 size=4; A0 input single size=4; A1 input single size=4; A2 input single size=4; A3 input single size=4; dDeltaX input single size=1; dDeltaY input single size=1; CosOfPsi input single size=1; SinOfPsi input single size=1; vRef input single size=1; error_right output single size=1; error_left output single size=1; pre_A3_2 output single size=1; pre_A2_2 output single size=1; pre_A1_2 output single size=1; pre_A0_2 output single size=1; pre_A3_3 output single size=1; pre_A2_3 output single size=1; pre_A1_3 output single size=1; pre_A0_3 output single size=1; pre_A3_2K1 input single size=1; pre_A2_2K1 input single size=1; pre_A1_2K1 input single size=1; pre_A0_2K1 input single size=1; pre_A3_3K1 input single size=1; pre_A2_3K1 input single size=1; pre_A1_3K1 input single size=1; pre_A0_3K1 input single size=1; pre_LineConfK1 input uint8 size=4; pre_LineConf output uint8 size=4
function [LeftOffset_b,RightOffset_b,error_right,error_left,pre_A3_2,pre_A2_2,pre_A1_2,pre_A0_2,...
    pre_A3_3,pre_A2_3,pre_A1_3,pre_A0_3,pre_LineConf] = ...
    LineTracker(LineUpdate,LineConf,A0,A1,A2,A3,...
    dDeltaX,dDeltaY,CosOfPsi,SinOfPsi,vRef,pre_A3_2K1,pre_A2_2K1,pre_A1_2K1,pre_A0_2K1,...
    pre_A3_3K1,pre_A2_3K1,pre_A1_3K1,pre_A0_3K1,pre_LineConfK1)

%%  当车道线更新时对比当前车道的右侧线和上一帧数据预测的车辆左侧线重合度判断是否发生左侧换道，右侧亦然
LeftOffset_b = false;
RightOffset_b = false;
error_right = single(3.5);
error_left = single(3.5);
pre_LineConf = LineConf;
t_Dist = max(single(15),vRef*1.8);
x = [0.05*t_Dist;0.3*t_Dist;0.6*t_Dist;t_Dist];
y2 = A3(2)*x.^3 + A2(2)*x.^2 + A1(2)*x + A0(2);
y3 = A3(3)*x.^3 + A2(3)*x.^2 + A1(3)*x + A0(3);
t_dx = x-dDeltaX;
t_dy2 = y2-dDeltaY;
t_dy3 = y3-dDeltaY;
TmpX2 = t_dx*CosOfPsi+t_dy2*SinOfPsi;
TmpY2 = -t_dx*SinOfPsi+t_dy2*CosOfPsi;
TmpX3 = t_dx*CosOfPsi+t_dy3*SinOfPsi;
TmpY3 = -t_dx*SinOfPsi+t_dy3*CosOfPsi;
[pre_A3_2,pre_A2_2,pre_A1_2,pre_A0_2] = pl(TmpX2,TmpY2);
[pre_A3_3,pre_A2_3,pre_A1_3,pre_A0_3] = pl(TmpX3,TmpY3);
if LineUpdate
    error_right = abs(A0(2)-pre_A0_3K1);
    error_left = abs(A0(3)-pre_A0_2K1);
    if (error_right<0.7 && pre_LineConfK1(3)>0 && LineConf(2)>0 && abs(57.3*(atan(A1(2))-atan(pre_A1_3K1)))<5)...
            ||(abs(error_left)>6 && pre_LineConfK1(2)>0 && LineConf(3)>0)||(LineConf(2)>0&&pre_LineConfK1(2)>0&&abs(A0(2))-abs(pre_A0_2)<-2)...
            ||(LineConf(3)>0&&pre_LineConfK1(3)>0&&abs(A0(3))-abs(pre_A0_3)>2)
        LeftOffset_b = false;
        RightOffset_b = true;
    elseif (error_left<0.7 && pre_LineConfK1(2)>0 && LineConf(3)>0 && abs(57.3*(atan(A1(3))-atan(pre_A1_2K1)))<5)...
            ||(abs(error_right)>6 && pre_LineConfK1(3)>0 && LineConf(2)>0)||(LineConf(2)>0&&pre_LineConfK1(2)>0&&abs(A0(2))-abs(pre_A0_2)>2)...
            ||(LineConf(3)>0&&pre_LineConfK1(3)>0&&abs(A0(3))-abs(pre_A0_3)<-2)
        LeftOffset_b = true;
        RightOffset_b = false;
    end
end

== matlab function PubIfDecisionLSM_MDL/Subsystem1/TargetLineCalc_20ms2/TargetLineCalc/TypeConf/RoadWidthCalc1 ==
  data: LeftType input uint8 size=1; LeftDLMType input; LeftDECELType input; RightType input uint8 size=1; RightDLMType input; RightDECELType input; Cnt1K1 input uint8 size=1; Cnt2K1 input uint8 size=1; LeftEn output boolean size=1; RightEn output boolean size=1; Cnt1 output uint8 size=1; Cnt2 output uint8 size=1
function [LeftEn,RightEn,Cnt1,Cnt2] = Delay(LeftType,LeftDLMType,LeftDECELType,RightType,RightDLMType,RightDECELType,Cnt1K1,Cnt2K1)
Cnt1 = max(Cnt1K1 - uint8(1),uint8(0));
Cnt2 = max(Cnt2K1 - uint8(1),uint8(0));
if LeftType==1||LeftType==6||(LeftType==3&&(LeftDLMType~=2||LeftDLMType~=4))||(LeftType==5&&(LeftDECELType~=2))
   Cnt1 = uint8(10); 
end
if RightType==1||RightType==6||(RightType==3&&(RightDLMType~=2||RightDLMType~=4))||(RightType==5&&(RightDECELType~=2))
   Cnt2 = uint8(10); 
end

if Cnt1>0
    LeftEn = false;
else
    LeftEn = true;
end

if Cnt2>0
    RightEn = false;
else
    RightEn = true;
end
end
